simulink model "DiagramaDeBloques_6"  (R2024b)
settings: Solver=VariableStepAuto  StartTime=0.0  StopTime=.01  RelTol=1e-3
settings Model: Creator=Charles
settings SolverCC: AlgebraicLoopSolver=TrustRegion
settings DataIOCC: ReturnWorkspaceOutputs=off
settings DebuggingCC: UnconnectedInputMsg=warning  UnconnectedOutputMsg=warning  UnconnectedLineMsg=warning  ArithmeticOperatorsInVariantConditions=warning
settings ModelReferenceCC: EnableRefExpFcnMdlSchedulingChecks=on
settings SFSimCC: SimUseLocalCustomCode=off  CustomCodeUndefinedFunction=UseInterfaceOnly
settings RTWCC: RTWUseLocalCustomCode=off  GPUComputeCapability=3.5

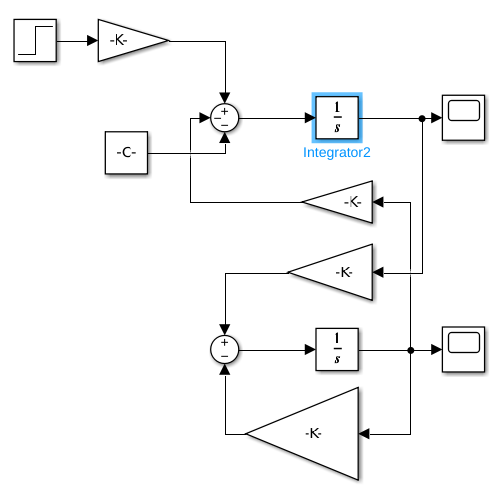
[thumbnail: Simulink's stored preview of the top-level diagram]
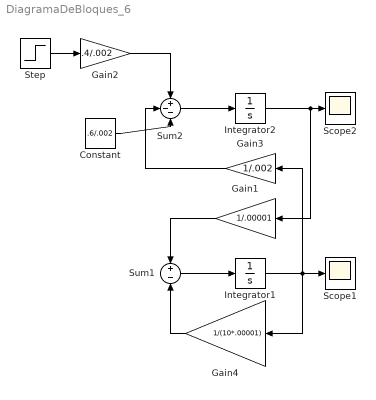
== system DiagramaDeBloques_6 ==
  Constant : Constant  Value=.6/.002
  Gain1 : Gain  Gain=1/.00001
  Gain2 : Gain  Gain=.4/.002
  Gain3 : Gain  Gain=1/.002
  Gain4 : Gain  Gain=1/(10*.00001)
  Integrator1 : Integrator
  Integrator2 : Integrator
  Scope1 : Scope
  Scope2 : Scope
  Step : Step  Time=0  After=32  SampleTime=0
  Sum1 : Sum  Inputs=+-
  Sum2 : Sum  Inputs=+--
  wires:
  Integrator1/1 -> Gain4/1, Gain3/1, Scope1/1
  Integrator2/1 -> Gain1/1, Scope2/1
  Step/1 -> Gain2/1
  Gain2/1 -> Sum2/1
  Sum2/1 -> Integrator2/1
  Sum1/1 -> Integrator1/1
  Gain3/1 -> Sum2/2
  Constant/1 -> Sum2/3
  Gain1/1 -> Sum1/1
  Gain4/1 -> Sum1/2
